simulink model "F_Simulacija_greske"  (R2016a)
settings: Solver=VariableStepAuto  StartTime=0.0  StopTime=100  RelTol=1e-3
libraries: simulink x3
settings Model: Creator=AmelT  LastModifiedBy=AmelT

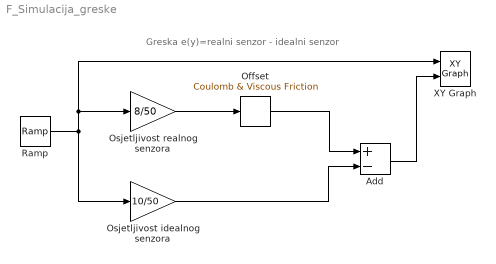
== system F_Simulacija_greske ==
  note: Greska e(y)=realni senzor - idealni senzor
  Add : Sum  Inputs=+-
  Offset : simulink/Discontinuities/Coulomb & Viscous Friction  offset=2  gain=1
  Osjetljivost idealnog senzora : Gain  Gain=10/50
  Osjetljivost realnog senzora : Gain  Gain=8/50
  Ramp : simulink/Sources/Ramp  slope=1  start=0  X0=-50
  XY Graph : simulink/Sinks/XY Graph  xmin=-50  xmax=50  ymin=-5  ymax=5  st=0
  wires:
  Ramp/1 -> Osjetljivost realnog senzora/1, XY Graph/1, Osjetljivost idealnog senzora/1
  Add/1 -> XY Graph/2
  Osjetljivost realnog senzora/1 -> Offset/1
  Osjetljivost idealnog senzora/1 -> Add/2
  Offset/1 -> Add/1
